simulink model "main_model"  (R2025a)
settings: Solver=VariableStepAuto  StartTime=0.0  StopTime=20  RelTol=1e-3
values from neighbouring files (symbols this model uses):
  E_up = 2*m*g*l    (= 4.508)    [LQR.m]
  g = 9.8    [LQR.m]
  I = (m*l^2)/3    (= 0.0766666666667)    [LQR.m]
  K = lqr(A, B, Q, R)    [LQR.m]
  l = 1    [LQR.m]
  M = 2.4    [LQR.m]
  m = 0.23    [LQR.m]
  n = 0.388    [LQR.m]
settings Model: Creator=Kush  LastModifiedBy=Kush

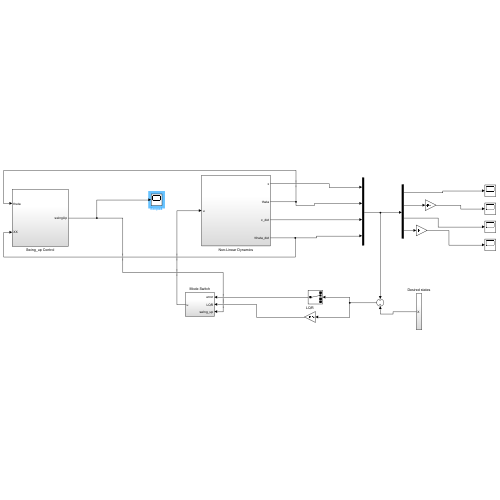
[thumbnail: Simulink's stored preview of the top-level diagram]
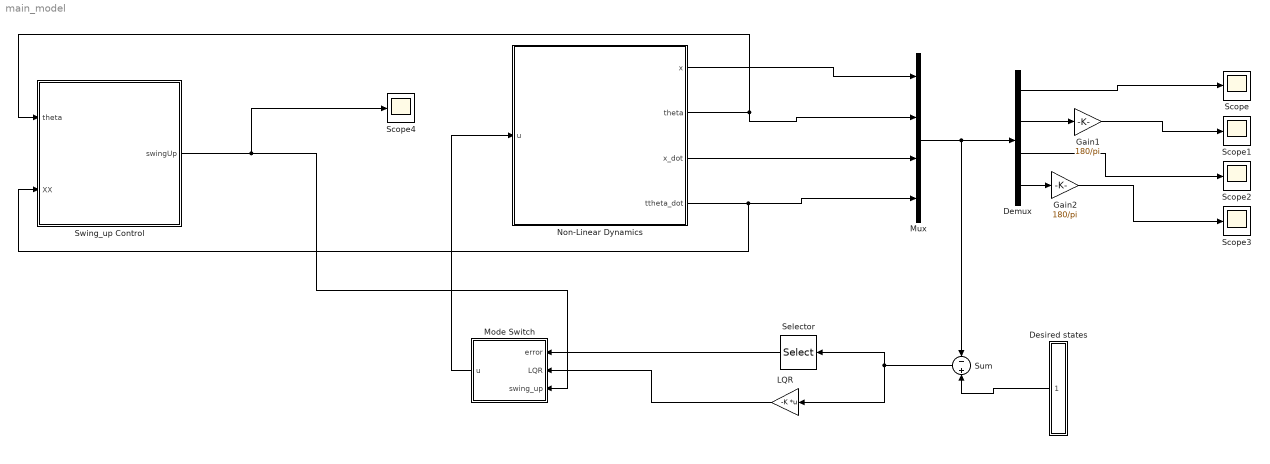
== system main_model ==
  Demux : Demux
  Desired states : Subsystem
  Gain1 : Gain  Gain=180/pi
  Gain2 : Gain  Gain=180/pi
  LQR : Gain  Gain=-K  Multiplication=Matrix(K*u)
  Mode Switch : Subsystem
  Mux : Mux
  Non-Linear Dynamics : Subsystem
  Scope{,1..4} (5 alike) : Scope
      Scope settings: ActiveDisplayYMinimum=-18.985593701736786  ActiveDisplayYMaximum=38.154497783084736
      Scope1 settings: ActiveDisplayYMinimum=-242.77041930858798  ActiveDisplayYMaximum=1005.6109272395425
      Scope2 settings: ActiveDisplayYMinimum=-19.835029952235818  ActiveDisplayYMaximum=19.259300249195693  DataLoggingVariableName=ScopeData2
      Scope3 settings: ActiveDisplayYMinimum=-1104.691035221203  ActiveDisplayYMaximum=1023.3336364371748  DataLoggingVariableName=ScopeData3
      Scope4 settings: SampleTime=0.01  ActiveDisplayYMinimum=-129.4679148729897  ActiveDisplayYMaximum=165.79884567352872  DataLoggingVariableName=ScopeData8
  Selector : Selector  InputPortWidth=4  IndexOptions=Index vector (dialog)  Indices=2  OutputSizes=1
  Sum : Sum  Inputs=-|+
  Swing_up Control : Subsystem
  wires:
  Mux/1 -> Demux/1, Sum/1
  Desired states/1(X) -> Sum/2
  Sum/1 -> LQR/1, Selector/1
  Selector/1 -> Mode Switch/1(error)
  LQR/1 -> Mode Switch/2(LQR)
  Demux/1 -> Scope/1
  Demux/3 -> Scope2/1
  Gain2/1 -> Scope3/1
  Demux/4 -> Gain2/1
  Non-Linear Dynamics/1(x) -> Mux/1
  Mode Switch/1(u) -> Non-Linear Dynamics/1(u)
  Non-Linear Dynamics/2(theta) -> Mux/2, Swing_up Control/1(theta)
  Non-Linear Dynamics/3(x_dot) -> Mux/3
  Non-Linear Dynamics/4(ttheta_dot) -> Swing_up Control/2(XX), Mux/4
  Demux/2 -> Gain1/1
  Gain1/1 -> Scope1/1
  Swing_up Control/1(swingUp) -> Scope4/1, Mode Switch/3(swing_up)

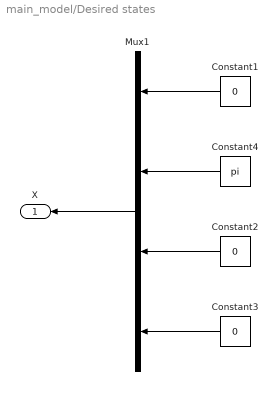
== system main_model/Desired states ==
  Constant1 : Constant  Value=0
  Constant2 : Constant  Value=0
  Constant3 : Constant  Value=0
  Constant4 : Constant  Value=pi
  Mux1 : Mux
  X : Outport
  wires:
  Constant2/1 -> Mux1/3
  Constant1/1 -> Mux1/1
  Constant3/1 -> Mux1/4
  Constant4/1 -> Mux1/2
  Mux1/1 -> X/1

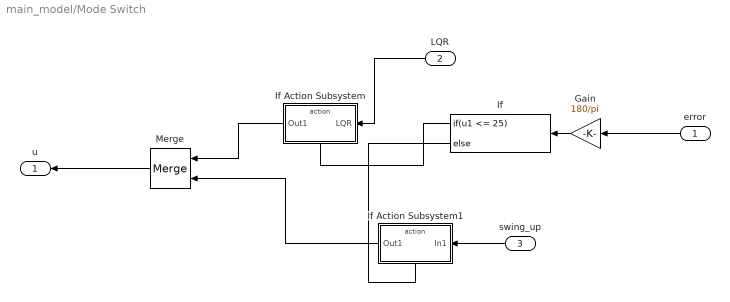
== system main_model/Mode Switch ==
  error : Inport
  LQR : Inport  Port=2
  swing_up : Inport  Port=3
  Gain : Gain  Gain=180/pi
  If : If  IfExpression=u1 <= 25
  If Action Subsystem : Subsystem  TreatAsAtomicUnit=on
  If Action Subsystem1 : Subsystem  TreatAsAtomicUnit=on
  Merge : Merge
  u : Outport
  wires:
  If Action Subsystem1/1(Out1) -> Merge/2
  Gain/1 -> If/1
  If/1 -> If Action Subsystem/Action
  swing_up/1 -> If Action Subsystem1/1(In1)
  error/1 -> Gain/1
  If Action Subsystem/1(Out1) -> Merge/1
  Merge/1 -> u/1
  If/2 -> If Action Subsystem1/Action
  LQR/1 -> If Action Subsystem/1(LQR)

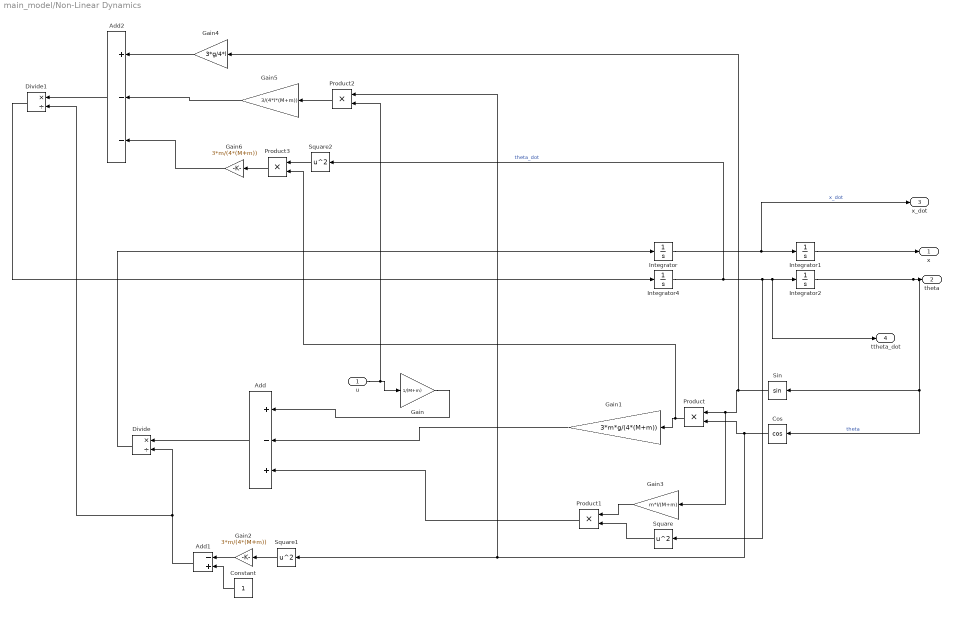
== system main_model/Non-Linear Dynamics ==
  u : Inport
  Add : Sum  Inputs=+-+
  Add1 : Sum  Inputs=-+
  Add2 : Sum  Inputs=+--
  Constant : Constant
  Cos : Trigonometry  Operator=cos
  Divide : Product  Inputs=*/
  Divide1 : Product  Inputs=*/
  Gain : Gain  Gain=1/(M+m)
  Gain1 : Gain  Gain=3*m*g/(4*(M+m))
  Gain2 : Gain  Gain=3*m/(4*(M+m))
  Gain3 : Gain  Gain=m*l/(M+m)
  Gain4 : Gain  Gain=3*g/4*l
  Gain5 : Gain  Gain=3/(4*l*(M+m))
  Gain6 : Gain  Gain=3*m/(4*(M+m))
  Integrator : Integrator
  Integrator1 : Integrator
  Integrator2 : Integrator  InitialCondition=1*(pi/180)
  Integrator4 : Integrator
  Product{,1..3} (4 alike) : Product
  Sin : Trigonometry
  Square : Math  Operator=square
  Square1 : Math  Operator=square
  Square2 : Math  Operator=square
  x : Outport
  theta : Outport  Port=2
  x_dot : Outport  Port=3
  ttheta_dot : Outport  Port=4
  wires:
  Integrator1/1 -> x/1
  Integrator2/1 -> Cos/1, Sin/1, theta/1  "theta"
  Integrator/1 -> x_dot/1, Integrator1/1  "x_dot"
  Integrator4/1 -> Square2/1, Square/1, ttheta_dot/1, Integrator2/1  "theta_dot"
  u/1 -> Product2/2, Gain/1
  Gain/1 -> Add/1
  Sin/1 -> Gain4/1, Gain3/1, Product/1
  Cos/1 -> Product2/1, Square1/1, Product/2
  Product/1 -> Product3/2, Gain1/1
  Gain1/1 -> Add/2
  Gain3/1 -> Product1/1
  Square/1 -> Product1/2
  Product1/1 -> Add/3
  Square1/1 -> Gain2/1
  Gain2/1 -> Add1/1
  Constant/1 -> Add1/2
  Add/1 -> Divide/1
  Add1/1 -> Divide1/2, Divide/2
  Divide/1 -> Integrator/1
  Gain4/1 -> Add2/1
  Product2/1 -> Gain5/1
  Gain5/1 -> Add2/2
  Square2/1 -> Product3/1
  Product3/1 -> Gain6/1
  Gain6/1 -> Add2/3
  Add2/1 -> Divide1/1
  Divide1/1 -> Integrator4/1

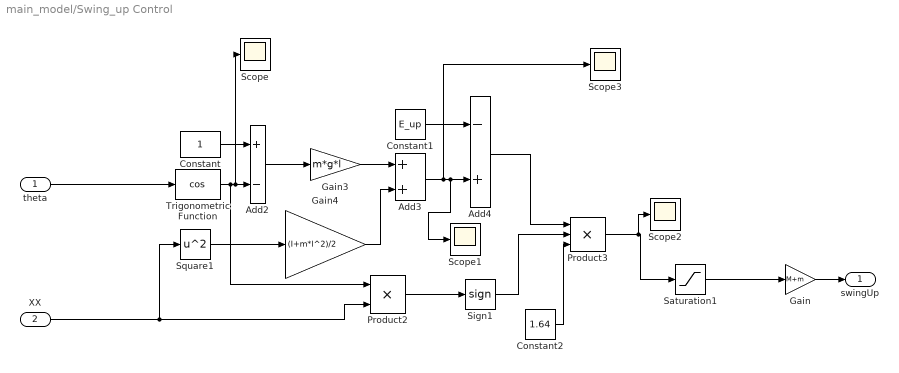
== system main_model/Swing_up Control ==
  theta : Inport
  XX : Inport  Port=2
  Add2 : Sum  Inputs=+-
  Add3 : Sum
  Add4 : Sum  Inputs=-+
  Constant : Constant
  Constant1 : Constant  Value=E_up
  Constant2 : Constant  Value=1.64
  Gain : Gain  Gain=M+m
  Gain3 : Gain  Gain=m*g*l
  Gain4 : Gain  Gain=(I+m*l^2)/2
  Product2 : Product
  Product3 : Product  Inputs=3
  Saturation1 : Saturate  UpperLimit=n*g  LowerLimit=-n*g
  Scope{,1..3} (4 alike) : Scope
      Scope settings: ActiveDisplayYMinimum=-1.8405365275633605  ActiveDisplayYMaximum=1.6894331863069394  DataLoggingVariableName=ScopeData4
      Scope1 settings: ActiveDisplayYMinimum=-0.1340268118869867  ActiveDisplayYMaximum=1.20685923819437  DataLoggingVariableName=ScopeData5
      Scope2 settings: ActiveDisplayYMinimum=-36.214502590661787  ActiveDisplayYMaximum=34.850449270926383  DataLoggingVariableName=ScopeData6
      Scope3 settings: ActiveDisplayYMinimum=-0.86836157808615266  ActiveDisplayYMaximum=5.9108943782313  DataLoggingVariableName=ScopeData7
  Sign1 : Signum
  Square1 : Math  Operator=square  SignedPower=on  RndMeth=Zero
  Trigonometric Function : Trigonometry  Operator=cos
  swingUp : Outport  VectorParamsAs1DForOutWhenUnconnected=off
  wires:
  XX/1 -> Product2/2, Square1/1
  Saturation1/1 -> Gain/1
  Trigonometric Function/1 -> Product2/1, Scope/1, Add2/2
  Product3/1 -> Scope2/1, Saturation1/1
  Square1/1 -> Gain4/1
  Add4/1 -> Product3/1
  Sign1/1 -> Product3/2
  Constant/1 -> Add2/1
  Constant1/1 -> Add4/1
  Gain4/1 -> Add3/2
  theta/1 -> Trigonometric Function/1
  Gain/1 -> swingUp/1
  Add2/1 -> Gain3/1
  Gain3/1 -> Add3/1
  Product2/1 -> Sign1/1
  Constant2/1 -> Product3/3
  Add3/1 -> Scope3/1, Scope1/1, Add4/2

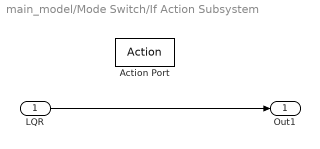
== system main_model/Mode Switch/If Action Subsystem ==
  LQR : Inport
  Action Port : ActionPort  ActionPortLabel=if(u1 <= 25)
  Out1 : Outport
  wires:
  LQR/1 -> Out1/1

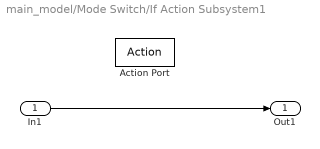
== system main_model/Mode Switch/If Action Subsystem1 ==
  In1 : Inport
  Action Port : ActionPort  ActionPortLabel=else
  Out1 : Outport
  wires:
  In1/1 -> Out1/1
